simulink model "inertia_simulink"  (R2024b)
settings: Solver=ode45  StartTime=0.0  StopTime=20  RelTol=1e-3
values from neighbouring files (symbols this model uses):
  Beq = 2.0e-6    (= 2e-06)    [Parameters_estimation.m]    (also in Real_time_parameter_estimation.m = (data.Beq_hat_pos + data.Beq_hat_neg)/2; data.m; real-time-estimation.mat = 1.22371676185e-06)
  degs2rpm = 60/360    (= 0.166666666667)    [Init.m]    (also in ModelParams.m; load_params_inertial_case.m)
  delta_est = 1/sqrt(2)    [Init.m]    (also in code.m; main.m)
  Kd = Kp * Td    [Init.m]    (also in code.m; main.m)
  Ki = Kp / Ti    [Init.m]    (also in code.m; main.m)
  Kp = deltak * cos(deltaphi)    [Init.m]    (also in code.m = deltak*cos(deltaphi); main.m = deltak*cos(deltaphi))
  pulse2deg = 360/ppr    (= 0.18)    [code.m]    (also in data.m)
  rpm2degs = 360/60    (= 6)    [Init.m]    (also in ModelParams.m; load_params_inertial_case.m)
  rpm2rads = 2*pi/60    (= 0.10471975512)    [Init.m]    (also in ModelParams.m; load_params_inertial_case.m)
  tau_sf = 1.0e-2    (= 0.01)    [Parameters_estimation.m]    (also in Real_time_parameter_estimation.m = (abs(data.tau_sf_pos)+abs(data.tau_sf_neg))/2; data.m; real-time-estimation.mat = 0.00570915114298)
  tl = 1/(3*wgc)    [Init.m]    (also in code.m = 1/cut_off; main.m = 1/cut_off)
  wc = 2*pi*20    (= 125.663706144)    [Init.m]    (also in code.m; main.m)
undefined symbols (not defined in the file or in its folder): gbox, mot
settings Model: Creator=lucag  LastModifiedBy=lucag

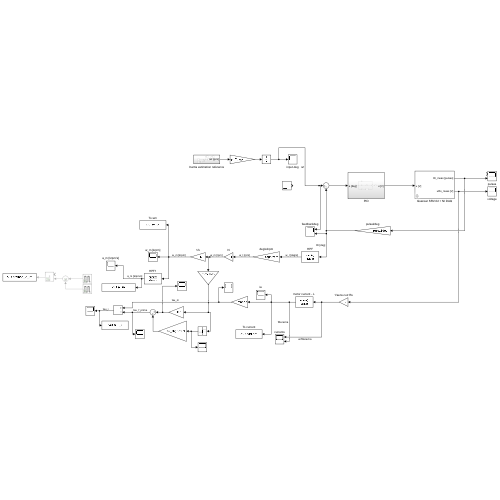
[thumbnail: Simulink's stored preview of the top-level diagram]
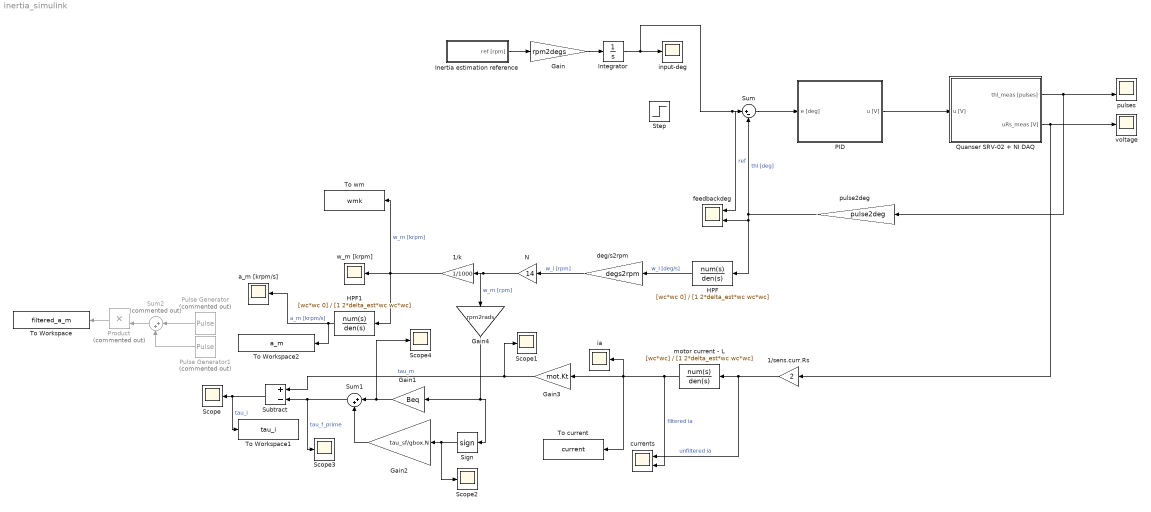
== system inertia_simulink ==
  1/k : Gain  Gain=1/1000
  1/sens.curr.Rs : Gain  Gain=2
  Gain : Gain  Gain=rpm2degs
  Gain1 : Gain  Gain=Beq
  Gain2 : Gain  Gain=tau_sf/gbox.N
  Gain3 : Gain  Gain=mot.Kt
  Gain4 : Gain  Gain=rpm2rads
  HPF : TransferFcn  Numerator=[wc*wc 0]  Denominator=[1 2*delta_est*wc wc*wc]
  HPF1 : TransferFcn  Numerator=[wc*wc 0]  Denominator=[1 2*delta_est*wc wc*wc]
  Inertia estimation reference : Subsystem
  Integrator : Integrator
  N : Gain  Gain=14
  PID : Subsystem
  Product : Product  Commented=on
  Pulse Generator : DiscretePulseGenerator  Commented=on  PulseType=Time based  Amplitude=6  PulseWidth=30  PhaseDelay=0.4
  Pulse Generator1 : DiscretePulseGenerator  Commented=on  PulseType=Time based  Amplitude=6  PulseWidth=30  PhaseDelay=1.4
  Quanser SRV-02 + NI DAQ : Subsystem  mask(Quanser SRV-02 (with inertial load) + NI DAQ){Ts=0.001, fricType=Coulomb + viscous}
      mask prompts: Ts "NI DAQ Sample Time:"; fricType "Friction model"
      mask help: Quanser SRV-02 (with inertial load) + NI DAQ model.
      mask init:
      | %%  Sensors data
      | 
      | %   shunt resistor
      | sens.curr.Rs = 0.5;                         %   resistance [Ohm]   
      | sens.curr.uRs_std = 0.01;                   %   voltage noise standard dev [V]                           
      | sens.curr.uRs_var = sens.curr.uRs_std^2;	%   voltage noise variance [V^2]
      | 
      | %   Hewlett-Packard HEDS-5540#A06 optical encoder
      | sens.enc.ppr = 500*4;                       %   pulses per rotation
      | sens.enc.pulse2deg = 360/sens.enc.ppr;      %   [pulses] -> [deg]
      | sens.enc.pulse2rad = 2*pi/sens.enc.ppr;     %   [pulses] -> [rad]
      | sens.enc.deg2pulse = sens.enc.ppr/360;      %   [deg] -> [pulses]
      | sens.enc.rad2pulse = sens.enc.ppr/2/pi;     %   [rad] -> [pulses]
      | 
      | 
      | %%  Data acquisition board (daq) data
      | 
      | %   NI PCI-6221 DAC data
      | daq.dac.bits = 16;                                  %   resolution (bits)
      | daq.dac.fs   = 10;                                  %   full scale 
      | daq.dac.q    = 2*daq.dac.fs/(2^daq.dac.bits-1);     %	quantization
      | 
      | %   NI PCI-6221 ADC data
      | daq.adc.bits = 16;                                  %   resolution (bits)
      | daq.adc.fs   = 10;                                  %   full scale (as set in SLDRT Analog Input block)
      | daq.adc.q    = 2*daq.adc.fs/(2^daq.adc.bits-1);     %   quantization
      mask Help:
      | Riccardo Antonello (antonello@dei.unipd.it)
      | 
      | April 24, 2020
      | 
      | Dept. of Information Engineering, University of Padova
      mask TypeOptions fricType: Coulomb + viscous | Karnopp
  Scope{,1..4} (5 alike) : Scope
  Sign : Signum  ZeroCross=off
  Step : Step  After=20  SampleTime=0
  Subtract : Sum  Inputs=+-
  Sum : Sum  Inputs=|+-
  Sum1 : Sum  Inputs=|++
  Sum2 : Sum  Commented=on  Inputs=|++
  To Workspace : ToWorkspace  VariableName=filtered_a_m  SaveFormat=Structure With Time  SampleTime=-1
  To Workspace1 : ToWorkspace  VariableName=tau_i  SaveFormat=Structure With Time  SampleTime=-1
  To Workspace2 : ToWorkspace  VariableName=a_m  SaveFormat=Structure With Time  SampleTime=-1
  To current : ToWorkspace  VariableName=current  SaveFormat=Structure With Time  SampleTime=-1
  To wm : ToWorkspace  VariableName=wmk  SaveFormat=Timeseries  SampleTime=-1
  a_m [krpm/s] : Scope
  currents : Scope  NumInputPorts=2
  deg/s2rpm : Gain  Gain=degs2rpm
  feedbackdeg : Scope  NumInputPorts=2
  ia : Scope
  input-deg : Scope
  "motor current - L " : TransferFcn  Numerator=[wc*wc]  Denominator=[1 2*delta_est*wc wc*wc]
  pulse2deg : Gain  Gain=pulse2deg
  pulses : Scope  NumInputPorts=2
  voltage : Scope
  w_m [krpm] : Scope
  wires:
  PID/1(u [V]) -> Quanser SRV-02 + NI DAQ/1(u [V])
  Inertia estimation reference/1(ref [rpm]) -> Gain/1
  Sum/1 -> PID/1(e [deg])
  HPF/1 -> deg/s2rpm/1  "w_l [deg/s]"
  Quanser SRV-02 + NI DAQ/1(thl_meas [pulses]) -> pulse2deg/1, pulses/2
  1/k/1 -> HPF1/1, To wm/1, w_m [krpm]/1  "w_m [krpm]"
  1/sens.curr.Rs/1 -> currents/1, "motor current - L "/1  "unfiltered ia"
  Integrator/1 -> feedbackdeg/1, Sum/1, input-deg/1  "ref"
  "motor current - L "/1 -> currents/2, To current/1, Gain3/1, ia/1  "filtered ia"
  deg/s2rpm/1 -> N/1  "w_l [rpm]"
  Quanser SRV-02 + NI DAQ/2(uRs_meas [V]) -> 1/sens.curr.Rs/1, voltage/1
  pulse2deg/1 -> HPF/1, feedbackdeg/2, Sum/2  "thl [deg]"
  Gain/1 -> Integrator/1
  HPF1/1 -> To Workspace2/1, a_m [krpm/s]/1  "a_m [krpm/s]"
  N/1 -> 1/k/1, Gain4/1  "w_m [rpm]"
  Gain1/1 -> Scope4/1, Sum1/1
  Sign/1 -> Scope2/1, Gain2/1
  Sum1/1 -> Scope3/1, Subtract/2  "tau_f_prime"
  Gain2/1 -> Sum1/2
  Gain3/1 -> Scope1/1, Subtract/1  "tau_m"
  Subtract/1 -> To Workspace1/1, Scope/1  "tau_i"
  Pulse Generator/1 -> Sum2/1
  Pulse Generator1/1 -> Sum2/2
  Sum2/1 -> Product/2
  Product/1 -> To Workspace/1
  Gain4/1 -> Gain1/1, Sign/1

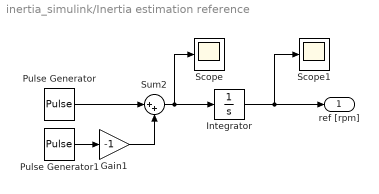
== system inertia_simulink/Inertia estimation reference ==
  Gain1 : Gain  Gain=-1
  Integrator : Integrator
  Pulse Generator : DiscretePulseGenerator  PulseType=Time based  Amplitude=450  PulseWidth=50
  Pulse Generator1 : DiscretePulseGenerator  PulseType=Time based  Amplitude=450  PulseWidth=50  PhaseDelay=1
  Scope : Scope
  Scope1 : Scope
  Sum2 : Sum  Inputs=|++
  ref [rpm] : Outport
  wires:
  Pulse Generator1/1 -> Gain1/1
  Gain1/1 -> Sum2/2
  Sum2/1 -> Integrator/1, Scope/1
  Pulse Generator/1 -> Sum2/1
  Integrator/1 -> Scope1/1, ref [rpm]/1

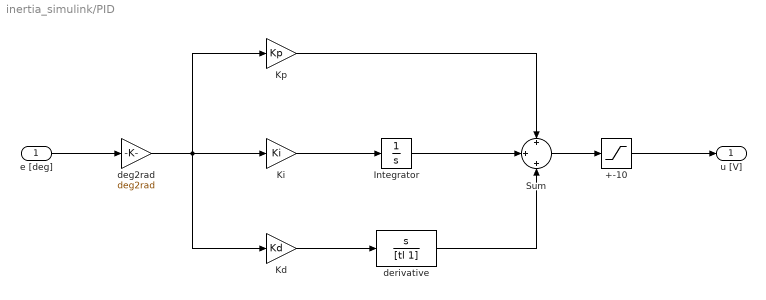
== system inertia_simulink/PID ==
  e [deg] : Inport
  +-10 : Saturate  UpperLimit=10  LowerLimit=-10
  Integrator : Integrator
  Kd : Gain  Gain=Kd
  Ki : Gain  Gain=Ki
  Kp : Gain  Gain=Kp
  Sum : Sum  Inputs=+|+|+
  deg2rad : Gain  Gain=deg2rad
  derivative : TransferFcn  Numerator=[1 0]  Denominator=[tl 1]
  u [V] : Outport
  wires:
  e [deg]/1 -> deg2rad/1
  deg2rad/1 -> Kd/1, Kp/1, Ki/1
  Ki/1 -> Integrator/1
  Kp/1 -> Sum/1
  Integrator/1 -> Sum/2
  Kd/1 -> derivative/1
  derivative/1 -> Sum/3
  Sum/1 -> +-10/1
  +-10/1 -> u [V]/1

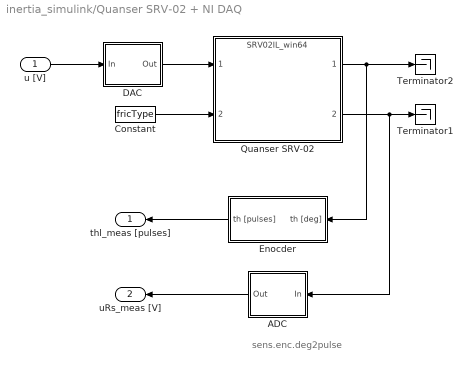
== system inertia_simulink/Quanser SRV-02 + NI DAQ ==
  note: sens.enc.deg2pulse
  u [V] : Inport
  ADC : Subsystem
  Constant : Constant  Value=fricType
  DAC : Subsystem
  Enocder : Subsystem
  Quanser SRV-02 : ModelReference  ModelNameDialog=SRV02IL_win64.slxp  ModelReferenceVersion=1.44  CopyOfModelProtected=on
  Terminator1 : Terminator
  Terminator2 : Terminator
  thl_meas [pulses] : Outport
  uRs_meas [V] : Outport  Port=2
  wires:
  Enocder/1(th [pulses]) -> thl_meas [pulses]/1
  ADC/1(Out) -> uRs_meas [V]/1
  DAC/1(Out) -> Quanser SRV-02/1
  Quanser SRV-02/2 -> ADC/1(In), Terminator1/1
  u [V]/1 -> DAC/1(In)
  Quanser SRV-02/1 -> Enocder/1(th [deg]), Terminator2/1
  Constant/1 -> Quanser SRV-02/2

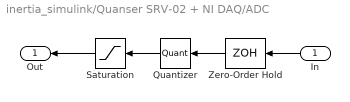
== system inertia_simulink/Quanser SRV-02 + NI DAQ/ADC ==
  In : Inport
  Quantizer : Quantizer  QuantizationInterval=daq.adc.q
  Saturation : Saturate  UpperLimit=daq.adc.fs  LowerLimit=-daq.adc.fs
  Zero-Order Hold : ZeroOrderHold  SampleTime=Ts
  Out : Outport
  wires:
  Saturation/1 -> Out/1
  In/1 -> Zero-Order Hold/1
  Quantizer/1 -> Saturation/1
  Zero-Order Hold/1 -> Quantizer/1

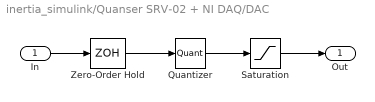
== system inertia_simulink/Quanser SRV-02 + NI DAQ/DAC ==
  In : Inport
  Quantizer : Quantizer  QuantizationInterval=daq.dac.q
  Saturation : Saturate  UpperLimit=daq.dac.fs  LowerLimit=-daq.dac.fs
  Zero-Order Hold : ZeroOrderHold  SampleTime=Ts
  Out : Outport
  wires:
  Quantizer/1 -> Saturation/1
  In/1 -> Zero-Order Hold/1
  Zero-Order Hold/1 -> Quantizer/1
  Saturation/1 -> Out/1

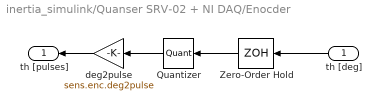
== system inertia_simulink/Quanser SRV-02 + NI DAQ/Enocder ==
  th [deg] : Inport
  Quantizer : Quantizer  QuantizationInterval=sens.enc.pulse2deg
  Zero-Order Hold : ZeroOrderHold  SampleTime=Ts
  deg2pulse : Gain  Gain=sens.enc.deg2pulse
  th [pulses] : Outport
  wires:
  Quantizer/1 -> deg2pulse/1
  th [deg]/1 -> Zero-Order Hold/1
  Zero-Order Hold/1 -> Quantizer/1
  deg2pulse/1 -> th [pulses]/1
